simulink model "q5_VAR"  (R2020b)
settings: Solver=ode4  StartTime=0.0  StopTime=SIM_TIME  FixedStep=STEP_SIZE  RelTol=1e-3
undefined symbols (not defined in the file): F_tf, seed, sigma_meas, T_s
libraries: cstblocks x2
settings Model: Creator=Theis  LastModifiedBy=Theis

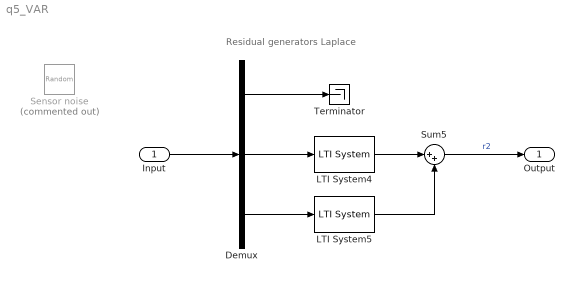
== system q5_VAR ==
  note: Residual generators
      | Laplace
  Input : Inport  PortDimensions=3
  Demux : Demux  Outputs=3
  LTI System4 : cstblocks/LTI System  sys=F_tf(2,2)  IC=[]
  LTI System5 : cstblocks/LTI System  sys=F_tf(2,3)  IC=[]
  Sensor noise : RandomNumber  Commented=on  Mean=zeros(3,1)  Variance=diag(sigma_meas^2)  Seed=seed  SampleTime=T_s
  Sum5 : Sum  Inputs=|++
  Terminator : Terminator
  Output : Outport  PortDimensions=1
  wires:
  Demux/1 -> Terminator/1
  Sum5/1 -> Output/1  "r2"
  LTI System5/1 -> Sum5/2
  LTI System4/1 -> Sum5/1
  Demux/3 -> LTI System5/1
  Demux/2 -> LTI System4/1
  Input/1 -> Demux/1
